simulink model "simulink_gazebo"  (R2023b)
settings: Solver=VariableStepAuto  StartTime=0.0  StopTime=10  RelTol=1e-3
undefined symbols (not defined in the file or in its folder): gray
libraries: robotgazebolib x2, visiongeotforms x2, deeplib x1
settings Model: Creator=Young  LastModifiedBy=Young

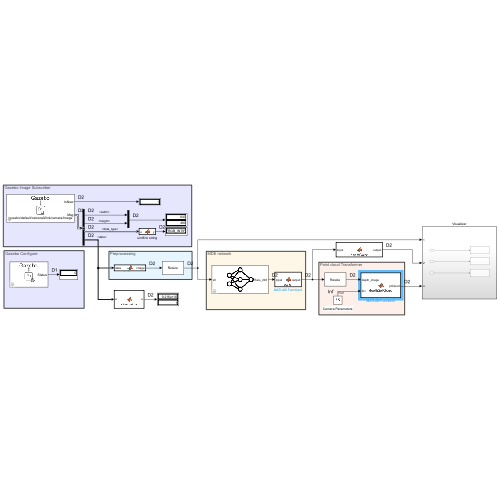
[thumbnail: Simulink's stored preview of the top-level diagram]
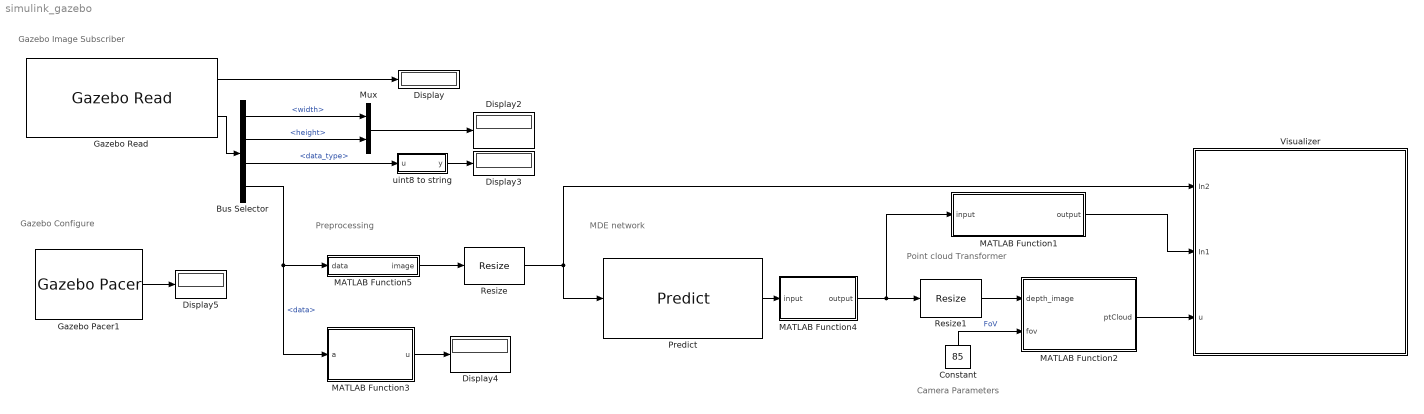
== system simulink_gazebo ==
  note: Gazebo Image Subscriber
  note: Point cloud Transformer
  note: MDE network
  note: Preprocessing
  note: Camera Parameters
  note: Gazebo Configure
  Bus Selector : BusSelector  OutputSignals=width,height,data_type,data
  Constant : Constant  Value=85  VectorParams1D=off
  Display{,2..5} (5 alike) : Display
  Gazebo Pacer1 : robotgazebolib/Gazebo Pacer  ResetBehavior=Reset Gazebo simulation time and scene  SampleTime=0.01
  Gazebo Read : robotgazebolib/Gazebo Read  topicSource=From Gazebo  topic=/gazebo/default/camera0/link/camera/image  messageType=gazebo_msgs/Image  sampleTime=1  fixedAxisBusStatus=off  jointAxisCount=2
  MATLAB Function1 : MATLAB Function  TreatAsAtomicUnit=on
  MATLAB Function2 : MATLAB Function  TreatAsAtomicUnit=on
  MATLAB Function3 : MATLAB Function  TreatAsAtomicUnit=on
  MATLAB Function4 : MATLAB Function  TreatAsAtomicUnit=on
  MATLAB Function5 : MATLAB Function  TreatAsAtomicUnit=on
  Mux : Mux  Inputs=2
  Predict : deeplib/Predict  Network=Network from MAT-file  NetworkFunction=squeezenet  NetworkFilePath=C:\Users\Young\Desktop\MATLAB_AI_COMP\model\net_MDE\net_trained_20230724.mat  MiniBatchSize=128  InputDataFormats={ 'x0', 'SSCB' }  Predictions=on  Activations={}  ForceInterpretedSim=off  EnableDLNetwork=on
  Resize : visiongeotforms/Resize  specify=Number of output rows and columns  rfactor=[200 150]  outCols=25  outRows=25  outRowsCols=[384 384]  interp_method=Bilinear  antialias=on  useROI=off  roiFlag=off  roundingMode=Nearest  overflowMode=on  prodOutputMode=Binary point scaling  prodOutputWordLength=32  prodOutputFracLength=10
  Resize1 : visiongeotforms/Resize  specify=Number of output rows and columns  rfactor=[200 150]  outCols=25  outRows=25  outRowsCols=[480 640]  interp_method=Bilinear  antialias=on  useROI=off  roiFlag=off  roundingMode=Nearest  overflowMode=on  prodOutputMode=Binary point scaling  prodOutputWordLength=32  prodOutputFracLength=10
  Visualizer : Subsystem
  uint8 to string : MATLAB Function  TreatAsAtomicUnit=on
  wires:
  Resize/1 -> Predict/1, Visualizer/1(In2)
  Predict/1 -> MATLAB Function4/1(input)
  MATLAB Function1/1(output) -> Visualizer/2(In1)
  Constant/1 -> MATLAB Function2/2(fov)  "FoV"
  Resize1/1 -> MATLAB Function2/1(depth_image)
  MATLAB Function2/1(ptCloud) -> Visualizer/3(u)
  MATLAB Function4/1(output) -> Resize1/1, MATLAB Function1/1(input)
  Gazebo Read/1 -> Display/1
  Gazebo Read/2 -> Bus Selector/1
  Mux/1 -> Display2/1
  Bus Selector/1 -> Mux/1  "<width>"
  Bus Selector/2 -> Mux/2  "<height>"
  Bus Selector/3 -> uint8 to string/1(u)  "<data_type>"
  uint8 to string/1(y) -> Display3/1
  Bus Selector/4 -> MATLAB Function5/1(data), MATLAB Function3/1(a)  "<data>"
  MATLAB Function3/1(u) -> Display4/1
  MATLAB Function5/1(image) -> Resize/1
  Gazebo Pacer1/1 -> Display5/1

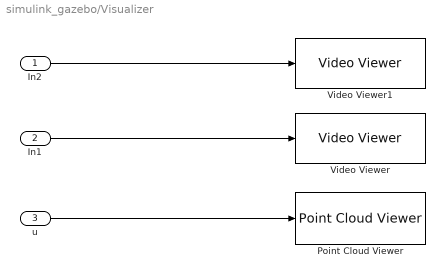
== system simulink_gazebo/Visualizer ==
  In2 : Inport
  In1 : Inport  Port=2
  u : Inport  Port=3
  Point Cloud Viewer : PointCloudViewer  FigPos=[254.6 859.6 419.2 538.4]
  Video Viewer : VideoViewer  colormapValue=gray(256)  FigPos=[3.4 609.2 245.6 280.8]
  Video Viewer1 : VideoViewer  colormapValue=gray(256)  FigPos=[3.4 577.2 245.6 256]
  wires:
  In1/1 -> Video Viewer/1
  u/1 -> Point Cloud Viewer/1
  In2/1 -> Video Viewer1/1

== matlab function simulink_gazebo/MATLAB Function4 ==
  data: input input; output output
function output = scaler(input)

p = [0 -0.0024 8.2238];
temp = p(2)*input + p(3);
output = 0.4838*temp + 3.129;

end

== matlab function simulink_gazebo/MATLAB Function1 ==
  data: input input; output output
function output = depthColor(input)

output = zeros([384 384 3]);

color_map = jet(256);
n_max = max(input(:));
n_min = min(input(:));

depth_data_colored = ind2rgb(uint8(256*(input - n_min)/(n_max - n_min)), color_map);
output = depth_data_colored;
end

== matlab function simulink_gazebo/MATLAB Function2 ==
  data: depth_image input; fov input; ptCloud output
function ptCloud = depth2ptCloud(depth_image, fov)
%fov, depth, resolution

pixels = 640*480; % from Resolution
crop = 10;
min_distance = 1;
max_distance = 6;   

cnt = 1;
pnt_pol = zeros([pixels,3]);
%이미지 사이즈가 정해지면 mask 형식으로 간단하게 계산하는 방법도 고려해보기
for i=1+crop:480-crop %세로
    for j=1+crop:640-crop %가로
        distance = depth_image(i,j);

        %% 기준각 pi/4
        angle_vert = -((2 * (i - 1) / (480 - 1)) - 1);  % 1 -> 1, 480 -> -1  
        angle_hor = -((2 * (j - 1) / (640 - 1)) - 1);  % 1 -> 1, 640 -> -1
        theta = pi/4 + deg2rad(fov/2)*angle_hor;
        rho = distance * cos(abs(deg2rad(fov/2)*angle_hor)); 
        z = distance * sin(abs(deg2rad(fov/2)*angle_vert)) *sign(angle_vert);    % 절대값 높이 * 부호
       
        % polar to cartsian coordinate
        [x,y,z] = pol2cart(theta,rho,z);
        if distance < max_distance  && distance > min_distance
        pnt_pol(cnt,:) = [x,y,z];
        end
        cnt = cnt+1;
    end
    
end 

ptCloud = pnt_pol;

== matlab function simulink_gazebo/MATLAB Function3 ==
  data: a input; u output
function u  = dimension(a)

u = size(a);


end

== matlab function simulink_gazebo/uint8 to string ==
  data: u input; y output
function y = convertUInt8VarSizeToString(u)

y = convertCharsToStrings(char(u'));

== matlab function simulink_gazebo/MATLAB Function5 ==
  data: data input; image output
function image = plotImage(data)

coder.extrinsic('imshow');
coder.extrinsic('helperPlotImage')

persistent h

if isempty(h)
    h = newplot(figure());
end

y = zeros(480, 640, 3, 'uint8');
if ~isempty(data) && ~isscalar(data)
    y(:) = helperPlotImage(data);
end
%imshow(y,'Parent',h);

image = im2double(y);
